simulink model "PowerFlow_TurboElectric_PartialTurboElectric"  (R2021b)
settings: Solver=FixedStepAuto  StartTime=0.0  StopTime=10.0  FixedStep=0.02  RelTol=1e-3
libraries: Lib_EMTAT x12, slpidlib x3
settings Model: Creator=sbianco1  LastModifiedBy=sbianco1
settings SolverCC: AlgebraicLoopSolver=TrustRegion
settings DebuggingCC: SFMachineParentedDataDiag=warning

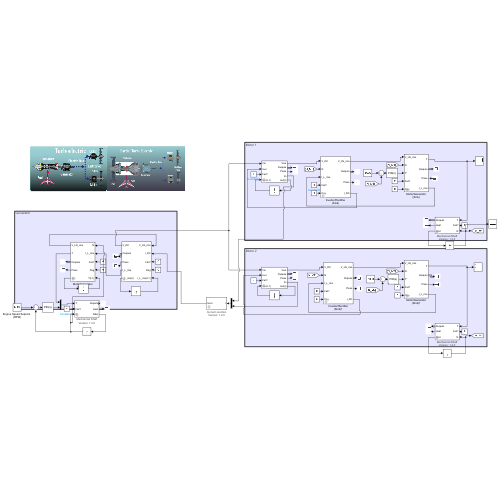
[thumbnail: Simulink's stored preview of the top-level diagram]
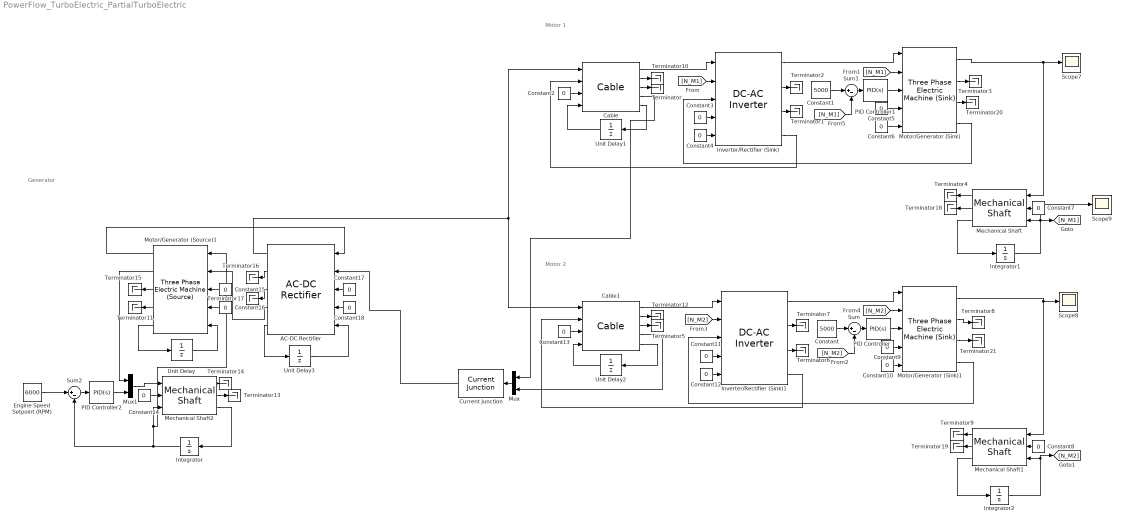
== system PowerFlow_TurboElectric_PartialTurboElectric ==
  note: Generator
  note: Motor 1
  note: Motor 2
  AC-DC Rectifier : Lib_EMTAT/Components/Power Flow/AC-DC Rectifier  X_C_VoltageInVec_M=[0 1000]  Y_C_RMSCurrentOutVec_M=[0 1000]  T_C_PowLossArray_M=0*ones(2)  FM=0  Plosslim=0
  Cable : Lib_EMTAT/Components/Power Flow/Cable  R=0.2
  Cable1 : Lib_EMTAT/Components/Power Flow/Cable  R=0.2
  Constant : Constant  Value=5000
  Constant1 : Constant  Value=5000
  Constant{2..18} (17 alike) : Constant  Value=0
  Current Junction : Lib_EMTAT/Components/Power Flow/Current Junction  Nb=2
      settings: AttributesFormatString=|
      | Current Junction
      | Version: %<LibraryVersion>
  Engine Speed Setpoint (RPM) : Constant  Value=6000
  Integrator : Integrator  InitialCondition=5000
  Integrator1 : Integrator
  Integrator2 : Integrator
  Inverter/Rectifier (Sink) : Lib_EMTAT/Components/Power Flow/DC-AC Inverter  X_C_VoltageInVec_M=[0 1000]  Y_C_RMSCurrentOutVec_M=[0 1000]  T_C_PowLossArray_M=100*ones(2)  K_e=0.0503  FM=0  Plosslim=0
  Inverter/Rectifier (Sink)1 : Lib_EMTAT/Components/Power Flow/DC-AC Inverter  X_C_VoltageInVec_M=[0 1000]  Y_C_RMSCurrentOutVec_M=[0 1000]  T_C_PowLossArray_M=100*ones(2)  K_e=0.0503  FM=0  Plosslim=0
  Mechanical Shaft : Lib_EMTAT/Components/Power Flow/Mechanical Shaft  J=0.01  B=0.001  Nb=1
      settings: AttributesFormatString=|
      | Mechanical Shaft
      | Version: %<LibraryVersion>
  Mechanical Shaft1 : Lib_EMTAT/Components/Power Flow/Mechanical Shaft  J=0.01  B=0.001  Nb=1
      settings: AttributesFormatString=|
      | Mechanical Shaft
      | Version: %<LibraryVersion>
  Mechanical Shaft2 : Lib_EMTAT/Components/Power Flow/Mechanical Shaft  J=0.1  B=0.01  Nb=2
      settings: AttributesFormatString=|
      | Mechanical Shaft
      | Version: %<LibraryVersion>
  Motor/Generator (Sink) : Lib_EMTAT/Components/Power Flow/Three Phase Electric Machine (Sink)  X_C_SpeedVec_M=[0 100 1000 5000]  Y_C_TorqueVec_M=[0 10 100 150]  T_C_EffArray_M=0.99*ones(4,4)  FM=0
  Motor/Generator (Sink)1 : Lib_EMTAT/Components/Power Flow/Three Phase Electric Machine (Sink)  X_C_SpeedVec_M=[0 100 1000 5000]  Y_C_TorqueVec_M=[0 10 100 150]  T_C_EffArray_M=0.99*ones(4,4)  FM=0
  Motor/Generator (Source)1 : Lib_EMTAT/Components/Power Flow/Three Phase Electric Machine (Source)  X_C_SpeedVec_M=[0 100 1000 5000]  Y_C_TorqueVec_M=[0 10 100 150]  T_C_EffArray_M=0.99*ones(4,4)  Ke=0.0503  FM=0
  Mux : Mux  Inputs=2
  Mux1 : Mux  Inputs=2
  PID Controller : slpidlib/PID Controller  Controller=PID  Form=Parallel  TimeDomain=Continuous-time  UseExternalTs=off  SampleTime=-1  IntegratorMethod=Forward Euler  FilterMethod=Forward Euler  ControllerParametersSource=internal  P=0.01  I=0.01  D=0  UseFilter=on  N=100  TunerSelectOption=Transfer Function Based (PID Tuner App)  InitialConditionSource=internal  InitialConditionForIntegrator=0  InitialConditionForFilter=0  DifferentiatorICPrevScaledInput=0  ExternalReset=none  TrackingMode=off  Kt=1  LimitOutput=off  SatLimitsSource=internal  UpperSaturationLimit=inf  LowerSaturationLimit=-inf  LinearizeAsGain=on  AntiWindupMode=none  Kb=1  POutMin=[]  POutMax=[]  IOutMin=[]  IOutMax=[]  DOutMin=[]  DOutMax=[]  NOutMin=[]  NOutMax=[]  SumOutMin=[]  SumOutMax=[]  SaturationOutMin=[]  SaturationOutMax=[]  PParamMin=[]  PParamMax=[]  IParamMin=[]  IParamMax=[]  DParamMin=[]  DParamMax=[]  NParamMin=[]  NParamMax=[]  KbParamMin=[]  KbParamMax=[]  KtParamMin=[]  KtParamMax=[]  KbOutMin=[]  KbOutMax=[]  KtOutMin=[]  KtOutMax=[]  IntegratorOutMin=[]  IntegratorOutMax=[]  FilterOutMin=[]  FilterOutMax=[]  SumI1OutMin=[]  SumI1OutMax=[]  SumI2OutMin=[]  SumI2OutMax=[]  SumI3OutMin=[]  SumI3OutMax=[]  SumI4OutMin=[]  SumI4OutMax=[]  SumDOutMin=[]  SumDOutMax=[]  DifferentiatorOutMin=[]  DifferentiatorOutMax=[]  FilterDiffOutCoefMin=[]  FilterDiffOutCoefMax=[]  ReciprocalOutMin=[]  ReciprocalOutMax=[]  SumDenOutMin=[]  SumDenOutMax=[]  SumNumOutMin=[]  SumNumOutMax=[]  DivideOutMin=[]  DivideOutMax=[]  UdiffTsProdOutMin=[]  UdiffTsProdOutMax=[]  NTsProdOutMin=[]  NTsProdOutMax=[]  UintegralTsProdOutMin=[]  UintegralTsProdOutMax=[]  UngainTsProdOutMin=[]  UngainTsProdOutMax=[]  IntegratorContinuousStateAttributes=''  IntegratorStateMustResolveToSignalObject=off  IntegratorRTWStateStorageClass=Auto  FilterContinuousStateAttributes=''  FilterStateMustResolveToSignalObject=off  FilterRTWStateStorageClass=Auto  ParallelPVariant=InternalParameters  IdealPVariant=Disabled  IVariant=InternalParameters  DVariant=InternalParameters  IntegratorVariant=Continuous  SatVariant=Disabled  AWVariant=Passthrough  PCopyVariant=Disabled  TRVariant=Disabled  FdbkBlocksVariant=Forward  IdealPFdbkVariant=Disabled  SatFdbkVariant=Disabled  DerivativeFilterVariant=ContFilter  NVariant=InternalParameters  NCopyVariant=Disabled  FilterICVariant=InternalICsFilter  IntegratorICVariant=InternalICs  ExternalResetVariant=Disabled  TRSumVariant=Passthrough  SumFdbkVariant=Disabled  SumVariant=Sum_PID  TsampFilterVariant=InternalTs  TsampNgainVariant=Passthrough  TsampIntegralVariant=Passthrough  ExternalSaturationOutDataTypeStr=Inherit: Same as second input
  PID Controller1 : slpidlib/PID Controller  Controller=PID  Form=Parallel  TimeDomain=Continuous-time  UseExternalTs=off  SampleTime=-1  IntegratorMethod=Forward Euler  FilterMethod=Forward Euler  ControllerParametersSource=internal  P=0.01  I=0.01  D=0  UseFilter=on  N=100  TunerSelectOption=Transfer Function Based (PID Tuner App)  InitialConditionSource=internal  InitialConditionForIntegrator=0  InitialConditionForFilter=0  DifferentiatorICPrevScaledInput=0  ExternalReset=none  TrackingMode=off  Kt=1  LimitOutput=off  SatLimitsSource=internal  UpperSaturationLimit=inf  LowerSaturationLimit=-inf  LinearizeAsGain=on  AntiWindupMode=none  Kb=1  POutMin=[]  POutMax=[]  IOutMin=[]  IOutMax=[]  DOutMin=[]  DOutMax=[]  NOutMin=[]  NOutMax=[]  SumOutMin=[]  SumOutMax=[]  SaturationOutMin=[]  SaturationOutMax=[]  PParamMin=[]  PParamMax=[]  IParamMin=[]  IParamMax=[]  DParamMin=[]  DParamMax=[]  NParamMin=[]  NParamMax=[]  KbParamMin=[]  KbParamMax=[]  KtParamMin=[]  KtParamMax=[]  KbOutMin=[]  KbOutMax=[]  KtOutMin=[]  KtOutMax=[]  IntegratorOutMin=[]  IntegratorOutMax=[]  FilterOutMin=[]  FilterOutMax=[]  SumI1OutMin=[]  SumI1OutMax=[]  SumI2OutMin=[]  SumI2OutMax=[]  SumI3OutMin=[]  SumI3OutMax=[]  SumI4OutMin=[]  SumI4OutMax=[]  SumDOutMin=[]  SumDOutMax=[]  DifferentiatorOutMin=[]  DifferentiatorOutMax=[]  FilterDiffOutCoefMin=[]  FilterDiffOutCoefMax=[]  ReciprocalOutMin=[]  ReciprocalOutMax=[]  SumDenOutMin=[]  SumDenOutMax=[]  SumNumOutMin=[]  SumNumOutMax=[]  DivideOutMin=[]  DivideOutMax=[]  UdiffTsProdOutMin=[]  UdiffTsProdOutMax=[]  NTsProdOutMin=[]  NTsProdOutMax=[]  UintegralTsProdOutMin=[]  UintegralTsProdOutMax=[]  UngainTsProdOutMin=[]  UngainTsProdOutMax=[]  IntegratorContinuousStateAttributes=''  IntegratorStateMustResolveToSignalObject=off  IntegratorRTWStateStorageClass=Auto  FilterContinuousStateAttributes=''  FilterStateMustResolveToSignalObject=off  FilterRTWStateStorageClass=Auto  ParallelPVariant=InternalParameters  IdealPVariant=Disabled  IVariant=InternalParameters  DVariant=InternalParameters  IntegratorVariant=Continuous  SatVariant=Disabled  AWVariant=Passthrough  PCopyVariant=Disabled  TRVariant=Disabled  FdbkBlocksVariant=Forward  IdealPFdbkVariant=Disabled  SatFdbkVariant=Disabled  DerivativeFilterVariant=ContFilter  NVariant=InternalParameters  NCopyVariant=Disabled  FilterICVariant=InternalICsFilter  IntegratorICVariant=InternalICs  ExternalResetVariant=Disabled  TRSumVariant=Passthrough  SumFdbkVariant=Disabled  SumVariant=Sum_PID  TsampFilterVariant=InternalTs  TsampNgainVariant=Passthrough  TsampIntegralVariant=Passthrough  ExternalSaturationOutDataTypeStr=Inherit: Same as second input
  PID Controller2 : slpidlib/PID Controller  Controller=PID  Form=Parallel  TimeDomain=Continuous-time  UseExternalTs=off  SampleTime=-1  IntegratorMethod=Forward Euler  FilterMethod=Forward Euler  ControllerParametersSource=internal  P=0.1  I=0.1  D=0  UseFilter=on  N=100  TunerSelectOption=Transfer Function Based (PID Tuner App)  InitialConditionSource=internal  InitialConditionForIntegrator=0  InitialConditionForFilter=0  DifferentiatorICPrevScaledInput=0  ExternalReset=none  TrackingMode=off  Kt=1  LimitOutput=off  SatLimitsSource=internal  UpperSaturationLimit=inf  LowerSaturationLimit=-inf  LinearizeAsGain=on  AntiWindupMode=none  Kb=1  POutMin=[]  POutMax=[]  IOutMin=[]  IOutMax=[]  DOutMin=[]  DOutMax=[]  NOutMin=[]  NOutMax=[]  SumOutMin=[]  SumOutMax=[]  SaturationOutMin=[]  SaturationOutMax=[]  PParamMin=[]  PParamMax=[]  IParamMin=[]  IParamMax=[]  DParamMin=[]  DParamMax=[]  NParamMin=[]  NParamMax=[]  KbParamMin=[]  KbParamMax=[]  KtParamMin=[]  KtParamMax=[]  KbOutMin=[]  KbOutMax=[]  KtOutMin=[]  KtOutMax=[]  IntegratorOutMin=[]  IntegratorOutMax=[]  FilterOutMin=[]  FilterOutMax=[]  SumI1OutMin=[]  SumI1OutMax=[]  SumI2OutMin=[]  SumI2OutMax=[]  SumI3OutMin=[]  SumI3OutMax=[]  SumI4OutMin=[]  SumI4OutMax=[]  SumDOutMin=[]  SumDOutMax=[]  DifferentiatorOutMin=[]  DifferentiatorOutMax=[]  FilterDiffOutCoefMin=[]  FilterDiffOutCoefMax=[]  ReciprocalOutMin=[]  ReciprocalOutMax=[]  SumDenOutMin=[]  SumDenOutMax=[]  SumNumOutMin=[]  SumNumOutMax=[]  DivideOutMin=[]  DivideOutMax=[]  UdiffTsProdOutMin=[]  UdiffTsProdOutMax=[]  NTsProdOutMin=[]  NTsProdOutMax=[]  UintegralTsProdOutMin=[]  UintegralTsProdOutMax=[]  UngainTsProdOutMin=[]  UngainTsProdOutMax=[]  IntegratorContinuousStateAttributes=''  IntegratorStateMustResolveToSignalObject=off  IntegratorRTWStateStorageClass=Auto  FilterContinuousStateAttributes=''  FilterStateMustResolveToSignalObject=off  FilterRTWStateStorageClass=Auto  ParallelPVariant=InternalParameters  IdealPVariant=Disabled  IVariant=InternalParameters  DVariant=InternalParameters  IntegratorVariant=Continuous  SatVariant=Disabled  AWVariant=Passthrough  PCopyVariant=Disabled  TRVariant=Disabled  FdbkBlocksVariant=Forward  IdealPFdbkVariant=Disabled  SatFdbkVariant=Disabled  DerivativeFilterVariant=ContFilter  NVariant=InternalParameters  NCopyVariant=Disabled  FilterICVariant=InternalICsFilter  IntegratorICVariant=InternalICs  ExternalResetVariant=Disabled  TRSumVariant=Passthrough  SumFdbkVariant=Disabled  SumVariant=Sum_PID  TsampFilterVariant=InternalTs  TsampNgainVariant=Passthrough  TsampIntegralVariant=Passthrough  ExternalSaturationOutDataTypeStr=Inherit: Same as second input
  Scope7 : Scope
  Scope8 : Scope
  Scope9 : Scope
  Sum : Sum  Inputs=|+-
  Sum1 : Sum  Inputs=|+-
  Sum2 : Sum  Inputs=|+-
  Terminator{,1..21} (22 alike) : Terminator
  Unit Delay : UnitDelay  InitialCondition=30  SampleTime=-1  HasFrameUpgradeWarning=on
  Unit Delay1 : UnitDelay  InitialCondition=56  SampleTime=-1  HasFrameUpgradeWarning=on
  Unit Delay2 : UnitDelay  SampleTime=-1  HasFrameUpgradeWarning=on
  Unit Delay3 : UnitDelay  InitialCondition=30  SampleTime=-1  HasFrameUpgradeWarning=on
  wires:
  Inverter/Rectifier (Sink)/1 -> Motor/Generator (Sink)/1
  Motor/Generator (Sink)/2 -> Terminator3/1
  Cable/1 -> Inverter/Rectifier (Sink)/1
  Inverter/Rectifier (Sink)/2 -> Terminator2/1
  Inverter/Rectifier (Sink)/3 -> Terminator1/1
  [N_M1] -> Motor/Generator (Sink)/2
  Motor/Generator (Sink)/1 -> Scope7/1, Mechanical Shaft/1
  [N_M1] -> Inverter/Rectifier (Sink)/2
  Motor/Generator (Sink)/4 -> Inverter/Rectifier (Sink)/3
  Inverter/Rectifier (Sink)/4 -> Cable/2
  Cable1/3 -> Terminator5/1
  Motor/Generator (Sink)1/4 -> Inverter/Rectifier (Sink)1/3
  Inverter/Rectifier (Sink)1/4 -> Cable1/2
  Inverter/Rectifier (Sink)1/3 -> Terminator6/1
  [N_M2] -> Motor/Generator (Sink)1/2
  [N_M2] -> Inverter/Rectifier (Sink)1/2
  Motor/Generator (Sink)1/1 -> Scope8/1, Mechanical Shaft1/1
  Motor/Generator (Sink)1/2 -> Terminator8/1
  Cable1/1 -> Inverter/Rectifier (Sink)1/1
  Inverter/Rectifier (Sink)1/1 -> Motor/Generator (Sink)1/1
  Inverter/Rectifier (Sink)1/2 -> Terminator7/1
  Motor/Generator (Source)1/1 -> AC-DC Rectifier/1
  AC-DC Rectifier/1 -> Cable/1, Cable1/1
  Motor/Generator (Source)1/3 -> Terminator15/1
  Motor/Generator (Source)1/4 -> Terminator11/1
  Cable/3 -> Terminator/1
  Cable/2 -> Terminator10/1
  Cable/4 -> Mux/1
  Cable1/2 -> Terminator12/1
  Constant/1 -> Sum/1
  [N_M2] -> Sum/2
  Sum/1 -> PID Controller/1
  PID Controller/1 -> Motor/Generator (Sink)1/3
  Sum1/1 -> PID Controller1/1
  [N_M1] -> Sum1/2
  Constant1/1 -> Sum1/1
  PID Controller1/1 -> Motor/Generator (Sink)/3
  AC-DC Rectifier/2 -> Terminator16/1
  AC-DC Rectifier/3 -> Terminator17/1
  Motor/Generator (Source)1/2 -> Mux1/1
  Current Junction/1 -> AC-DC Rectifier/2
  Mux/1 -> Current Junction/1
  Cable1/4 -> Mux/2
  Motor/Generator (Source)1/5 -> Unit Delay/1
  Unit Delay/1 -> Motor/Generator (Source)1/5
  AC-DC Rectifier/4 -> Motor/Generator (Source)1/2
  Integrator/1 -> Sum2/2, Mechanical Shaft2/3, Motor/Generator (Source)1/1
  Cable/5 -> Unit Delay1/1
  Unit Delay1/1 -> Cable/4
  Cable1/5 -> Unit Delay2/1
  Unit Delay2/1 -> Cable1/4
  Integrator1/1 -> Scope9/1, [N_M1], Mechanical Shaft/3
  Integrator2/1 -> Mechanical Shaft1/3, [N_M2]
  Mux1/1 -> Mechanical Shaft2/1
  PID Controller2/1 -> Mux1/2
  Engine Speed Setpoint (RPM)/1 -> Sum2/1
  Sum2/1 -> PID Controller2/1
  AC-DC Rectifier/5 -> Unit Delay3/1
  Mechanical Shaft/1 -> Terminator4/1
  Mechanical Shaft/2 -> Terminator18/1
  Mechanical Shaft/3 -> Integrator1/1
  Constant2/1 -> Cable/3
  Constant3/1 -> Inverter/Rectifier (Sink)/4
  Constant4/1 -> Inverter/Rectifier (Sink)/5
  Constant5/1 -> Motor/Generator (Sink)/4
  Constant6/1 -> Motor/Generator (Sink)/5
  Constant7/1 -> Mechanical Shaft/2
  Mechanical Shaft1/1 -> Terminator9/1
  Mechanical Shaft1/2 -> Terminator19/1
  Mechanical Shaft1/3 -> Integrator2/1
  Constant8/1 -> Mechanical Shaft1/2
  Constant9/1 -> Motor/Generator (Sink)1/4
  Constant10/1 -> Motor/Generator (Sink)1/5
  Motor/Generator (Sink)1/3 -> Terminator21/1
  Constant11/1 -> Inverter/Rectifier (Sink)1/4
  Constant12/1 -> Inverter/Rectifier (Sink)1/5
  Constant13/1 -> Cable1/3
  Mechanical Shaft2/1 -> Terminator14/1
  Mechanical Shaft2/2 -> Terminator13/1
  Mechanical Shaft2/3 -> Integrator/1
  Constant14/1 -> Mechanical Shaft2/2
  Constant15/1 -> Motor/Generator (Source)1/3
  Constant16/1 -> Motor/Generator (Source)1/4
  Unit Delay3/1 -> AC-DC Rectifier/5
  Constant17/1 -> AC-DC Rectifier/3
  Constant18/1 -> AC-DC Rectifier/4
  Motor/Generator (Sink)/3 -> Terminator20/1
